simulink model "serialtransmittest_electrogarm"  (R2017b)
settings: Solver=FixedStepAuto  StartTime=0.0  StopTime=64  FixedStep=0.001  RelTol=1e-3  EnableMultiTasking=on
undefined symbols (not defined in the file): A0, A1, D13, PTB2, PTB3, PTD1
libraries: frdmk64flib x4, etargetslib x1
settings Model: ExtModeTrigDuration=5  Creator=brydoa1  LastModifiedBy=puerstee
settings OptimizationCC: PassReuseOutputArgsAs=Individual arguments  MaxStackSize=64
settings DebuggingCC: ParameterTunabilityLossMsg=error
settings HardwareCC: ProdBitPerPointer=32  ProdBitPerSizeT=32  ProdBitPerPtrDiffT=32  ProdLargestAtomicInteger=Long  ProdLargestAtomicFloat=Double  ProdWordSize=32  ProdHWDeviceType=ARM Compatible->ARM Cortex
settings SFSimCC: MATLABDynamicMemAlloc=off
settings RTWCC: SystemTargetFile=ert.tlc  HardwareBoard=NXP FRDM-K64F  TemplateMakefile=ert_default_tmf  GenerateReport=on  Toolchain=GNU Tools for ARM Embedded Processors  IncludeHyperlinkInReport=on  LaunchReport=on  GenerateTraceInfo=on  GenerateTraceReport=on  GenerateTraceReportSl=on  GenerateTraceReportSf=on  GenerateTraceReportEml=on
settings CodeAppCC: ForceParamTrailComments=on  IgnoreCustomStorageClasses=off  OperatorAnnotations=on  SimulinkDataObjDesc=on  SFDataObjDesc=on  InsertBlockDesc=on

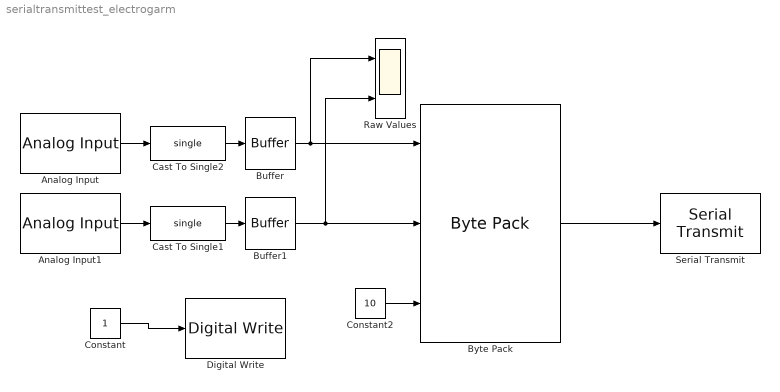
== system serialtransmittest_electrogarm ==
  Analog Input : frdmk64flib/Analog Input  Whichpin=PTB3 (A1)  SampleTime=0.002
      settings: SourceProductName=Simulink Coder Support Package for NXP FRDM-K64F Board
  Analog Input1 : frdmk64flib/Analog Input  Whichpin=PTB2 (A0)  SampleTime=0.002
      settings: SourceProductName=Simulink Coder Support Package for NXP FRDM-K64F Board
  Buffer : Buffer  N=100  OutputFrames=off
  Buffer1 : Buffer  N=100  OutputFrames=off
  Byte Pack : etargetslib/Byte Pack  datatypes={'single','single','uint8'}  byteAlign=1
  Cast To Single1 : DataTypeConversion  OutDataTypeStr=single
  Cast To Single2 : DataTypeConversion  OutDataTypeStr=single
  Constant : Constant
  Constant2 : Constant  Value=10  OutDataTypeStr=uint8  SampleTime=0.2
  Digital Write : frdmk64flib/Digital Write  Whichpin=PTD1 (D13)
      settings: SourceProductName=Simulink Coder Support Package for NXP FRDM-K64F Board
  "Raw Values " : Scope  NumInputPorts=2
  Serial Transmit : frdmk64flib/Serial Transmit  SCIModule=0  Baudrate=uint32(9600)  Parity=None  StopBits=1  HardwareFlowControl=None  ByteOrder=LittleEndian  BlockingMode=on  OutputStatus=off
      settings: SourceProductName=Simulink Coder Support Package for NXP FRDM-K64F Board
  wires:
  Constant2/1 -> Byte Pack/3
  Buffer/1 -> "Raw Values "/1, Byte Pack/1
  Cast To Single2/1 -> Buffer/1
  Analog Input/1 -> Cast To Single2/1
  Buffer1/1 -> "Raw Values "/2, Byte Pack/2
  Analog Input1/1 -> Cast To Single1/1
  Cast To Single1/1 -> Buffer1/1
  Byte Pack/1 -> Serial Transmit/1
  Constant/1 -> Digital Write/1
